simulink model "Simple_Model_Packaging_4_1"  (R2022b)
settings: Solver=VariableStepAuto  StartTime=0.0  StopTime=0.03  RelTol=1e-3
InitFcn:
  | Parameter_Initialize_4
undefined symbols (not defined in the file or in its folder): gcbh, model, rcfiltgaincompat, rsgenpoly
libraries: dspobslib x11, commdigbbndpm3 x6, commdigbbndam3 x6, simulink x5, commblkintrlv2 x4, commfilt2 x4, commsynccomp2 x3, commblkcod2 x2, commrandsrc3 x2, commseqgen3 x2, commchan3 x1, dspsigops x1
(part 2 of 2)

== system Simple_Model_Packaging_4_1/帧序列识别器/Subsystem2 ==
  In1 : Inport
  Constant : Constant
  Constant1 : Constant  Value=-1
  If : If  IfExpression=u1 ==1
  If Action Subsystem : Subsystem  TreatAsAtomicUnit=on
  If Action Subsystem1 : Subsystem  TreatAsAtomicUnit=on
  Merge : Merge
  Out1 : Outport
  wires:
  If Action Subsystem1/1(Out1) -> Merge/2
  If/2 -> If Action Subsystem1/Action
  In1/1 -> If/1
  If Action Subsystem/1(Out1) -> Merge/1
  If/1 -> If Action Subsystem/Action
  Merge/1 -> Out1/1
  Constant1/1 -> If Action Subsystem1/1(In1)
  Constant/1 -> If Action Subsystem/1(In1)

== system Simple_Model_Packaging_4_1/帧序列识别器/Subsystem3 ==
  In1 : Inport
  Constant : Constant
  Constant1 : Constant  Value=-1
  If : If  IfExpression=u1 ==2
  If Action Subsystem : Subsystem  TreatAsAtomicUnit=on
  If Action Subsystem1 : Subsystem  TreatAsAtomicUnit=on
  Merge : Merge
  Out1 : Outport
  wires:
  Constant/1 -> If Action Subsystem/1(In1)
  Constant1/1 -> If Action Subsystem1/1(In1)
  Merge/1 -> Out1/1
  If/1 -> If Action Subsystem/Action
  If Action Subsystem/1(Out1) -> Merge/1
  In1/1 -> If/1
  If/2 -> If Action Subsystem1/Action
  If Action Subsystem1/1(Out1) -> Merge/2

== system Simple_Model_Packaging_4_1/帧序列识别器/Subsystem4 ==
  In1 : Inport
  Constant : Constant
  Constant1 : Constant  Value=-1
  If : If  IfExpression=u1 ==3
  If Action Subsystem : Subsystem  TreatAsAtomicUnit=on
  If Action Subsystem1 : Subsystem  TreatAsAtomicUnit=on
  Merge : Merge
  Out1 : Outport
  wires:
  If Action Subsystem1/1(Out1) -> Merge/2
  If/2 -> If Action Subsystem1/Action
  In1/1 -> If/1
  If Action Subsystem/1(Out1) -> Merge/1
  If/1 -> If Action Subsystem/Action
  Merge/1 -> Out1/1
  Constant1/1 -> If Action Subsystem1/1(In1)
  Constant/1 -> If Action Subsystem/1(In1)

== system Simple_Model_Packaging_4_1/帧序列识别器/Subsystem5 ==
  In1 : Inport
  Constant : Constant
  Constant1 : Constant  Value=-1
  If : If  IfExpression=u1 ==2
  If Action Subsystem : Subsystem  TreatAsAtomicUnit=on
  If Action Subsystem1 : Subsystem  TreatAsAtomicUnit=on
  Merge : Merge
  Out1 : Outport
  wires:
  Constant/1 -> If Action Subsystem/1(In1)
  Constant1/1 -> If Action Subsystem1/1(In1)
  Merge/1 -> Out1/1
  If/1 -> If Action Subsystem/Action
  If Action Subsystem/1(Out1) -> Merge/1
  In1/1 -> If/1
  If/2 -> If Action Subsystem1/Action
  If Action Subsystem1/1(Out1) -> Merge/2

== system Simple_Model_Packaging_4_1/帧序列识别器/Subsystem6 ==
  In1 : Inport
  Constant : Constant
  Constant1 : Constant  Value=-1
  If : If  IfExpression=u1 ==1
  If Action Subsystem : Subsystem  TreatAsAtomicUnit=on
  If Action Subsystem1 : Subsystem  TreatAsAtomicUnit=on
  Merge : Merge
  Out1 : Outport
  wires:
  If Action Subsystem1/1(Out1) -> Merge/2
  If/2 -> If Action Subsystem1/Action
  In1/1 -> If/1
  If Action Subsystem/1(Out1) -> Merge/1
  If/1 -> If Action Subsystem/Action
  Merge/1 -> Out1/1
  Constant1/1 -> If Action Subsystem1/1(In1)
  Constant/1 -> If Action Subsystem/1(In1)

== system Simple_Model_Packaging_4_1/帧序列识别器/Subsystem7 ==
  In1 : Inport
  Constant : Constant
  Constant1 : Constant  Value=-1
  If : If  IfExpression=u1 ==3
  If Action Subsystem : Subsystem  TreatAsAtomicUnit=on
  If Action Subsystem1 : Subsystem  TreatAsAtomicUnit=on
  Merge : Merge
  Out1 : Outport
  wires:
  Constant/1 -> If Action Subsystem/1(In1)
  Constant1/1 -> If Action Subsystem1/1(In1)
  Merge/1 -> Out1/1
  If/1 -> If Action Subsystem/Action
  If Action Subsystem/1(Out1) -> Merge/1
  In1/1 -> If/1
  If/2 -> If Action Subsystem1/Action
  If Action Subsystem1/1(Out1) -> Merge/2

== system Simple_Model_Packaging_4_1/帧序列识别器/Triggered Subsystem ==
  y3_SS : Inport
  Trigger : TriggerPort  TriggerType=falling  VariantControl=(inherit)
  Out1 : Outport
  wires:
  y3_SS/1 -> Out1/1

== system Simple_Model_Packaging_4_1/信源基带解调/Baseband Signal Selector Rx/If Action Subsystem1 ==
  In1 : Inport
  Action Port : ActionPort  ActionPortLabel=elseif(u1 == 2)
  M-PSK Demodulator Baseband : commdigbbndpm3/M-PSK Demodulator Baseband  M=model.user_defined.Rectangular_QAM_Modulator_Baseband.M_Number  OutType=Integer  DecType=Hard decision  VarSource=Dialog  Variance=1  Dec=Gray  Mapping=[0:7]  Ph=0  outDtype1=Inherit via internal rule  outDtype2=Inherit via internal rule  derotateFactorWordLen=16  derotateFactorDataTypeStr=Inherit: Same word length as input  derotateFactorLastDataTypeStr=Inherit: Same word length as input
  Out1 : Outport
  wires:
  In1/1 -> M-PSK Demodulator Baseband/1
  M-PSK Demodulator Baseband/1 -> Out1/1  "REData"

== system Simple_Model_Packaging_4_1/信源基带解调/Baseband Signal Selector Rx/If Action Subsystem4 ==
  In1 : Inport
  Action Port : ActionPort  ActionPortLabel=if(u1 == 1)
  Rectangular QAM Demodulator Baseband : commdigbbndam3/Rectangular QAM Demodulator Baseband  M=model.user_defined.Rectangular_QAM_Modulator_Baseband.M_Number  OutType=Integer  DecType=Hard decision  VarSource=Dialog  Variance=1  Dec=Gray  Mapping=[0:15]  PowType=Min. distance between symbols  MinDist=model.parameter.Rectangular_QAM_Demodulator_Baseband.Minimum_distance  AvgPow=1  PeakPow=1  Ph=0  outDtype1=Inherit via internal rule  outDtype2=Inherit via internal rule  derotateFactorWordLen=16  derotateFactorDataTypeStr=Inherit: Same word length as input  derotateFactorLastDataTypeStr=Inherit: Same word length as input  denormFactorWordLen=16  denormFactorDataTypeStr=Inherit: Same word length as input  denormFactorLastDataTypeStr=Inherit: Same word length as input  prodOutWordLen=32  prodOutOverflowMode=Wrap  prodOutRoundingMode=Floor  prodOutOvFlMode=off  prodOutOvFlModeLastStrValue=off  sumWordLen=32
  Out1 : Outport
  wires:
  In1/1 -> Rectangular QAM Demodulator Baseband/1
  Rectangular QAM Demodulator Baseband/1 -> Out1/1  "REData"

== system Simple_Model_Packaging_4_1/信源基带解调/Baseband Signal Selector Rx/If Action Subsystem5 ==
  In1 : Inport
  Action Port : ActionPort  ActionPortLabel=else
  Rectangular QAM Demodulator Baseband : commdigbbndam3/Rectangular QAM Demodulator Baseband  M=model.user_defined.Rectangular_QAM_Modulator_Baseband.M_Number  OutType=Integer  DecType=Hard decision  VarSource=Dialog  Variance=1  Dec=Gray  Mapping=[0:15]  PowType=Min. distance between symbols  MinDist=2  AvgPow=1  PeakPow=1  Ph=0  outDtype1=Inherit via internal rule  outDtype2=Inherit via internal rule  derotateFactorWordLen=16  derotateFactorDataTypeStr=Inherit: Same word length as input  derotateFactorLastDataTypeStr=Inherit: Same word length as input  denormFactorWordLen=16  denormFactorDataTypeStr=Inherit: Same word length as input  denormFactorLastDataTypeStr=Inherit: Same word length as input  prodOutWordLen=32  prodOutOverflowMode=Wrap  prodOutRoundingMode=Floor  prodOutOvFlMode=off  prodOutOvFlModeLastStrValue=off  sumWordLen=32
  Out1 : Outport
  wires:
  In1/1 -> Rectangular QAM Demodulator Baseband/1
  Rectangular QAM Demodulator Baseband/1 -> Out1/1

== system Simple_Model_Packaging_4_1/信源部分基带调制/Baseband Signal Selector Tx/If Action Subsystem1 ==
  In1 : Inport
  Action Port : ActionPort  ActionPortLabel=elseif(u1 == 2)
  M-PSK Modulator Baseband : commdigbbndpm3/M-PSK Modulator Baseband  M=model.user_defined.Rectangular_QAM_Modulator_Baseband.M_Number  InType=Integer  Enc=Gray  Mapping=[0:7]  Ph=0  outDtype=double  outWordLen=16  outUDDataType=sfix(16)  outFracLenMode=Best precision  outFracLen=15  outDataTypeStr=double  outLastDataTypeStr=double
  Out1 : Outport
  wires:
  M-PSK Modulator Baseband/1 -> Out1/1
  In1/1 -> M-PSK Modulator Baseband/1

== system Simple_Model_Packaging_4_1/信源部分基带调制/Baseband Signal Selector Tx/If Action Subsystem4 ==
  In1 : Inport
  Action Port : ActionPort  ActionPortLabel=if(u1 == 1)
  Rectangular QAM Modulator Baseband : commdigbbndam3/Rectangular QAM Modulator Baseband  M=model.user_defined.Rectangular_QAM_Modulator_Baseband.M_Number  InType=Integer  Enc=Gray  Mapping=[0:15]  PowType=Min. distance between symbols  MinDist=model.parameter.Rectangular_QAM_Modulator_Baseband.Minimum_distance  AvgPow=1  PeakPow=1  Ph=0  outDtype=double  outWordLen=16  outUDDataType=sfix(16)  outFracLenMode=Best precision  outFracLen=15  outDataTypeStr=double  outLastDataTypeStr=double
      settings: LibrarySourceBlock=|
      | commhdldigbbndam/Rectangular QAM
      | Modulator
      | Baseband
  Out1 : Outport
  wires:
  Rectangular QAM Modulator Baseband/1 -> Out1/1
  In1/1 -> Rectangular QAM Modulator Baseband/1

== system Simple_Model_Packaging_4_1/信源部分基带调制/Baseband Signal Selector Tx/If Action Subsystem5 ==
  In1 : Inport
  Action Port : ActionPort  ActionPortLabel=else
  Rectangular QAM Modulator Baseband1 : commdigbbndam3/Rectangular QAM Modulator Baseband  M=model.user_defined.Rectangular_QAM_Modulator_Baseband.M_Number  InType=Integer  Enc=Gray  Mapping=[0:15]  PowType=Min. distance between symbols  MinDist=2  AvgPow=1  PeakPow=1  Ph=0  outDtype=double  outWordLen=16  outUDDataType=sfix(16)  outFracLenMode=Best precision  outFracLen=15  outDataTypeStr=double  outLastDataTypeStr=double
      settings: LibrarySourceBlock=|
      | commhdldigbbndam/Rectangular QAM
      | Modulator
      | Baseband
  Out1 : Outport
  wires:
  In1/1 -> Rectangular QAM Modulator Baseband1/1
  Rectangular QAM Modulator Baseband1/1 -> Out1/1

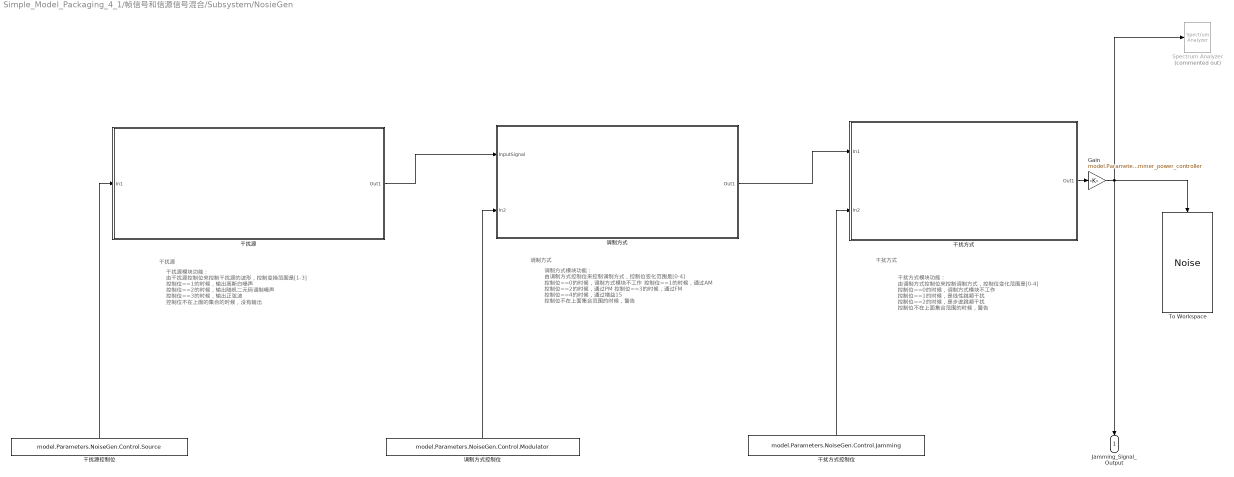
== system Simple_Model_Packaging_4_1/帧信号和信源信号混合/Subsystem/NosieGen ==
  note: 干扰方式模块功能：
      | 由调制方式控制位来控制调制方式，控制位变化范围是[0-4]
      | 控制位==0的时候，调制方式模块不工作
      | 控制位==1的时候，是线性跳频干扰
      | 控制位==2的时候，是步进跳频干扰
      | 控制位不在上面集合范围的时候，警告
  note: 干扰源模块功能：
      | 由干扰源控制位来控制干扰源的波形，控制变换范围是[1-3]
      | 控制位==1的时候，输出高斯白噪声
      | 控制位==2的时候，输出随机二元码调制噪声
      | 控制位==3的时候，输出正弦波
      | 控制位不在上面的集合的时候，没有输出
  note: 调制方式模块功能：
      | 由调制方式控制位来控制调制方式，控制位变化范围是[0-4]
      | 控制位==0的时候，调制方式模块不工作
      | 控制位==1的时候，通过AM
      | 控制位==2的时候，通过PM
      | 控制位==3的时候，通过FM
      | 控制位==4的时候，通过增益15
      | 控制位不在上面集合范围的时候，警告
  note: 干扰方式
  note: 干扰源
  note: 调制方式
  Gain : Gain  Gain=model.Parameters.jammer_power_controller
  Spectrum Analyzer : SpectrumAnalyzer  Commented=on
  To Workspace : ToWorkspace  VariableName=Noise  SaveFormat=Timeseries  SampleTime=-1
  干扰方式 : Subsystem
  干扰方式控制位 : Constant  Value=model.Parameters.NoiseGen.Control.Jamming  SampleTime=Inf
  干扰源 : Subsystem
  干扰源控制位 : Constant  Value=model.Parameters.NoiseGen.Control.Source  SampleTime=Inf
  调制方式 : Subsystem
  调制方式控制位 : Constant  Value=model.Parameters.NoiseGen.Control.Modulator  SampleTime=Inf
  Jamming_Signal_Output : Outport
  wires:
  干扰方式/1(Out1) -> Gain/1
  调制方式/1(Out1) -> 干扰方式/1(In1)
  干扰源/1(Out1) -> 调制方式/1(InputSignal)
  干扰方式控制位/1 -> 干扰方式/2(In2)
  干扰源控制位/1 -> 干扰源/1(In1)
  调制方式控制位/1 -> 调制方式/2(In2)
  Gain/1 -> To Workspace/1, Jamming_Signal_Output/1, Spectrum Analyzer/1

== system Simple_Model_Packaging_4_1/帧序列识别器/Subsystem/If Action Subsystem ==
  In1 : Inport
  Action Port : ActionPort  ActionPortLabel=if(u1 ==0)
  Out1 : Outport
  wires:
  In1/1 -> Out1/1

== system Simple_Model_Packaging_4_1/帧序列识别器/Subsystem/If Action Subsystem1 ==
  In1 : Inport
  Action Port : ActionPort  ActionPortLabel=else
  Out1 : Outport
  wires:
  In1/1 -> Out1/1

== system Simple_Model_Packaging_4_1/帧序列识别器/Subsystem1/If Action Subsystem ==
  In1 : Inport
  Action Port : ActionPort  ActionPortLabel=if(u1 ==3)
  Out1 : Outport
  wires:
  In1/1 -> Out1/1

== system Simple_Model_Packaging_4_1/帧序列识别器/Subsystem1/If Action Subsystem1 ==
  In1 : Inport
  Action Port : ActionPort  ActionPortLabel=else
  Out1 : Outport
  wires:
  In1/1 -> Out1/1

== system Simple_Model_Packaging_4_1/帧序列识别器/Subsystem2/If Action Subsystem ==
  In1 : Inport
  Action Port : ActionPort  ActionPortLabel=if(u1 ==1)
  Out1 : Outport
  wires:
  In1/1 -> Out1/1

== system Simple_Model_Packaging_4_1/帧序列识别器/Subsystem2/If Action Subsystem1 ==
  In1 : Inport
  Action Port : ActionPort  ActionPortLabel=else
  Out1 : Outport
  wires:
  In1/1 -> Out1/1

== system Simple_Model_Packaging_4_1/帧序列识别器/Subsystem3/If Action Subsystem ==
  In1 : Inport
  Action Port : ActionPort  ActionPortLabel=if(u1 ==2)
  Out1 : Outport
  wires:
  In1/1 -> Out1/1

== system Simple_Model_Packaging_4_1/帧序列识别器/Subsystem3/If Action Subsystem1 ==
  In1 : Inport
  Action Port : ActionPort  ActionPortLabel=else
  Out1 : Outport
  wires:
  In1/1 -> Out1/1

== system Simple_Model_Packaging_4_1/帧序列识别器/Subsystem4/If Action Subsystem ==
  In1 : Inport
  Action Port : ActionPort  ActionPortLabel=if(u1 ==3)
  Out1 : Outport
  wires:
  In1/1 -> Out1/1

== system Simple_Model_Packaging_4_1/帧序列识别器/Subsystem4/If Action Subsystem1 ==
  In1 : Inport
  Action Port : ActionPort  ActionPortLabel=else
  Out1 : Outport
  wires:
  In1/1 -> Out1/1

== system Simple_Model_Packaging_4_1/帧序列识别器/Subsystem5/If Action Subsystem ==
  In1 : Inport
  Action Port : ActionPort  ActionPortLabel=if(u1 ==2)
  Out1 : Outport
  wires:
  In1/1 -> Out1/1

== system Simple_Model_Packaging_4_1/帧序列识别器/Subsystem5/If Action Subsystem1 ==
  In1 : Inport
  Action Port : ActionPort  ActionPortLabel=else
  Out1 : Outport
  wires:
  In1/1 -> Out1/1

== system Simple_Model_Packaging_4_1/帧序列识别器/Subsystem6/If Action Subsystem ==
  In1 : Inport
  Action Port : ActionPort  ActionPortLabel=if(u1 ==1)
  Out1 : Outport
  wires:
  In1/1 -> Out1/1

== system Simple_Model_Packaging_4_1/帧序列识别器/Subsystem6/If Action Subsystem1 ==
  In1 : Inport
  Action Port : ActionPort  ActionPortLabel=else
  Out1 : Outport
  wires:
  In1/1 -> Out1/1

== system Simple_Model_Packaging_4_1/帧序列识别器/Subsystem7/If Action Subsystem ==
  In1 : Inport
  Action Port : ActionPort  ActionPortLabel=if(u1 ==3)
  Out1 : Outport
  wires:
  In1/1 -> Out1/1

== system Simple_Model_Packaging_4_1/帧序列识别器/Subsystem7/If Action Subsystem1 ==
  In1 : Inport
  Action Port : ActionPort  ActionPortLabel=else
  Out1 : Outport
  wires:
  In1/1 -> Out1/1

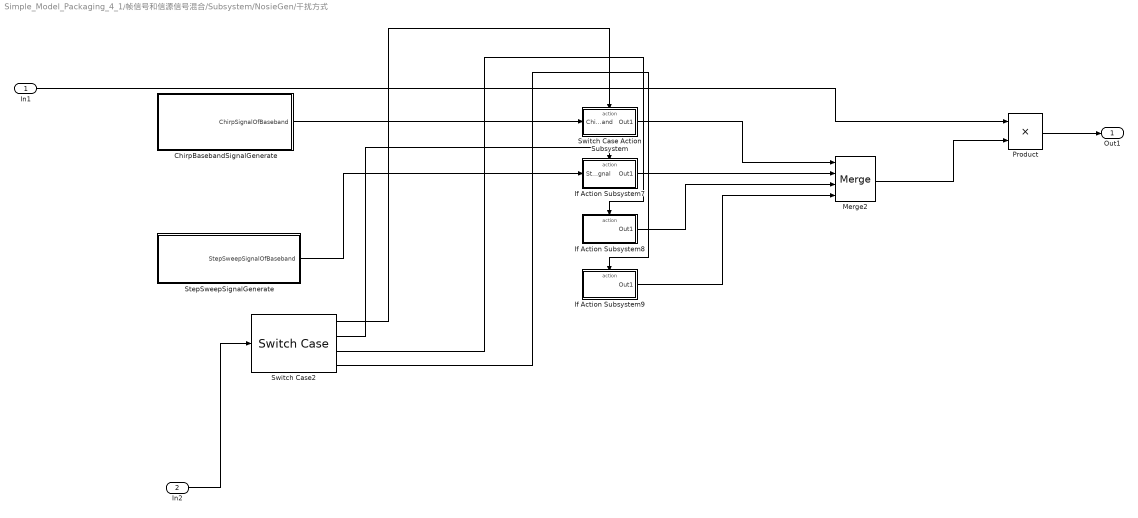
== system Simple_Model_Packaging_4_1/帧信号和信源信号混合/Subsystem/NosieGen/干扰方式 ==
  In1 : Inport
  In2 : Inport  Port=2
  ChirpBasebandSignalGenerate : Subsystem
      settings: AttributesFormatString=|
      | 线性调频模块：线性调频公式(y=exp(2*pi*(f_min*t+0.5*k_chirp*t^2)))
      | 输入参数：
      | 1. f_min,为线性调频信号的起始频率
      | 2.f_max为线性调频信号的终止频率
      | 3.T_chirp为线性调频信号的调频时间
      | 斜率k_sweep = (f_min-f_max)/T_chirp
  If Action Subsystem7 : Subsystem  TreatAsAtomicUnit=on
  If Action Subsystem8 : Subsystem  TreatAsAtomicUnit=on
  If Action Subsystem9 : Subsystem  TreatAsAtomicUnit=on
  Merge2 : Merge  Inputs=4
  Product : Product
  StepSweepSignalGenerate : Subsystem
  Switch Case Action Subsystem : Subsystem  TreatAsAtomicUnit=on
  Switch Case2 : SwitchCase  CaseConditions={1,2,3}
  Out1 : Outport
  wires:
  If Action Subsystem9/1(Out1) -> Merge2/4
  Switch Case Action Subsystem/1(Out1) -> Merge2/1
  If Action Subsystem8/1(Out1) -> Merge2/3
  Switch Case2/3 -> If Action Subsystem8/Action
  Switch Case2/1 -> Switch Case Action Subsystem/Action
  Switch Case2/2 -> If Action Subsystem7/Action
  Switch Case2/4 -> If Action Subsystem9/Action
  ChirpBasebandSignalGenerate/1(ChirpSignalOfBaseband) -> Switch Case Action Subsystem/1(ChirpSignalOfBaseband)
  If Action Subsystem7/1(Out1) -> Merge2/2
  Merge2/1 -> Product/2
  Product/1 -> Out1/1
  In1/1 -> Product/1
  In2/1 -> Switch Case2/1
  StepSweepSignalGenerate/1(StepSweepSignalOfBaseband) -> If Action Subsystem7/1(StepSweepSignal)

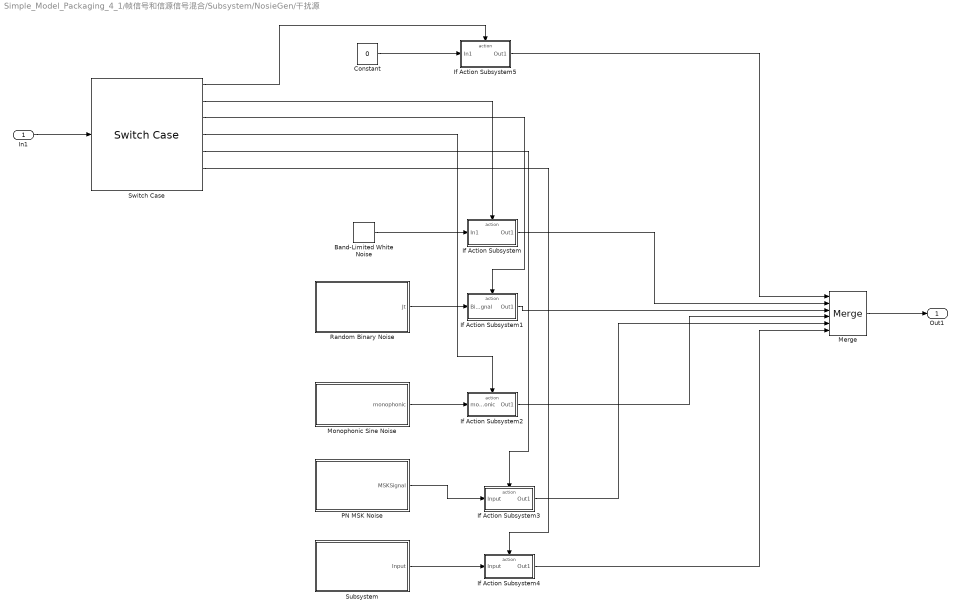
== system Simple_Model_Packaging_4_1/帧信号和信源信号混合/Subsystem/NosieGen/干扰源 ==
  In1 : Inport
  Band-Limited White Noise : simulink/Sources/Band-Limited White Noise  Cov=model.Parameters.NoiseGen.GaussPower  Ts=model.Parameters.NoiseGen.NoiseTs  seed=model.Parameters.NoiseGen.GaussSeed
  Constant : Constant  Value=0  SampleTime=model.Parameters.NoiseGen.NoiseTs
  If Action Subsystem : Subsystem  TreatAsAtomicUnit=on
  If Action Subsystem1 : Subsystem  TreatAsAtomicUnit=on
  If Action Subsystem2 : Subsystem  TreatAsAtomicUnit=on
  If Action Subsystem3 : Subsystem  TreatAsAtomicUnit=on
  If Action Subsystem4 : Subsystem  TreatAsAtomicUnit=on
  If Action Subsystem5 : Subsystem  TreatAsAtomicUnit=on
  Merge : Merge  Inputs=6
  Monophonic Sine Noise : Subsystem
  PN MSK Noise : Subsystem
  Random Binary Noise : Subsystem
  Subsystem : Subsystem
  Switch Case : SwitchCase  CaseConditions={0,1,2,3,4,5}
  Out1 : Outport
  wires:
  Switch Case/3 -> If Action Subsystem1/Action
  If Action Subsystem2/1(Out1) -> Merge/4
  Band-Limited White Noise/1 -> If Action Subsystem/1(In1)
  If Action Subsystem1/1(Out1) -> Merge/3
  Random Binary Noise/1(Jt) -> If Action Subsystem1/1(Binary_Random_Signal)
  Switch Case/4 -> If Action Subsystem2/Action
  Switch Case/2 -> If Action Subsystem/Action
  Merge/1 -> Out1/1
  In1/1 -> Switch Case/1
  Monophonic Sine Noise/1(monophonic) -> If Action Subsystem2/1(monophonic)
  Switch Case/5 -> If Action Subsystem3/Action
  If Action Subsystem3/1(Out1) -> Merge/5
  If Action Subsystem/1(Out1) -> Merge/2
  PN MSK Noise/1(MSKSignal) -> If Action Subsystem3/1(Input)
  Switch Case/6 -> If Action Subsystem4/Action
  Subsystem/1(Input) -> If Action Subsystem4/1(Input)
  If Action Subsystem4/1(Out1) -> Merge/6
  Switch Case/1 -> If Action Subsystem5/Action
  Constant/1 -> If Action Subsystem5/1(In1)
  If Action Subsystem5/1(Out1) -> Merge/1

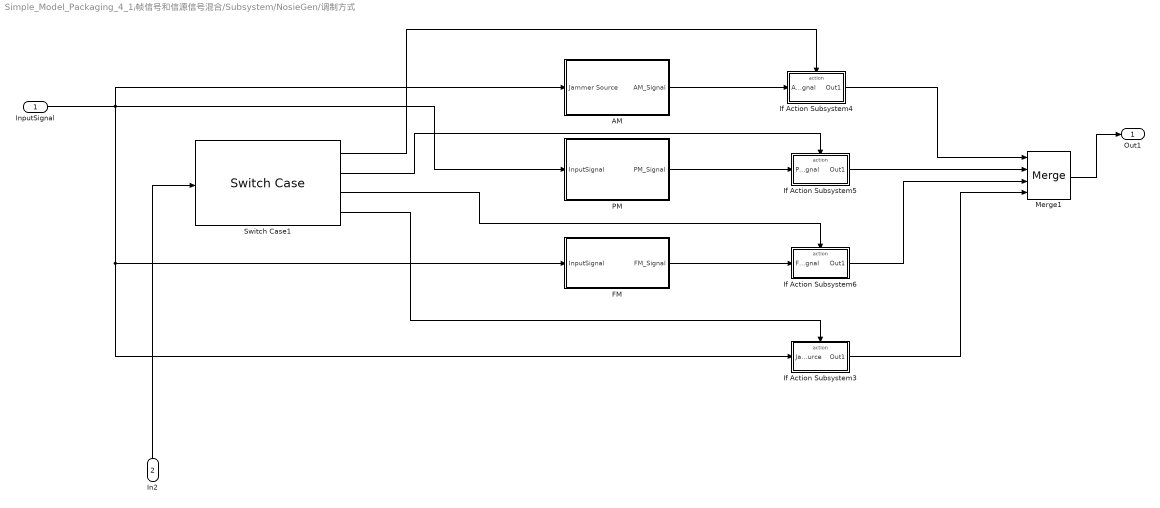
== system Simple_Model_Packaging_4_1/帧信号和信源信号混合/Subsystem/NosieGen/调制方式 ==
  InputSignal : Inport
  In2 : Inport  Port=2
  AM : Subsystem
  FM : Subsystem
  If Action Subsystem3 : Subsystem  TreatAsAtomicUnit=on
  If Action Subsystem4 : Subsystem  TreatAsAtomicUnit=on
  If Action Subsystem5 : Subsystem  TreatAsAtomicUnit=on
  If Action Subsystem6 : Subsystem  TreatAsAtomicUnit=on
  Merge1 : Merge  Inputs=4
  PM : Subsystem
  Switch Case1 : SwitchCase  CaseConditions={1,2,3}
  Out1 : Outport
  wires:
  In2/1 -> Switch Case1/1
  PM/1(PM_Signal) -> If Action Subsystem5/1(PM_Signal)
  Merge1/1 -> Out1/1
  If Action Subsystem3/1(Out1) -> Merge1/4
  If Action Subsystem6/1(Out1) -> Merge1/3
  If Action Subsystem5/1(Out1) -> Merge1/2
  InputSignal/1 -> AM/1(Jammer Source), FM/1(InputSignal), If Action Subsystem3/1(Jammer Source), PM/1(InputSignal)
  AM/1(AM_Signal) -> If Action Subsystem4/1(AM_Signal)
  Switch Case1/2 -> If Action Subsystem5/Action
  Switch Case1/3 -> If Action Subsystem6/Action
  Switch Case1/1 -> If Action Subsystem4/Action
  If Action Subsystem4/1(Out1) -> Merge1/1
  FM/1(FM_Signal) -> If Action Subsystem6/1(FM_Signal)
  Switch Case1/4 -> If Action Subsystem3/Action

== system Simple_Model_Packaging_4_1/帧信号和信源信号混合/Subsystem/NosieGen/干扰方式/ChirpBasebandSignalGenerate ==
  note: 线性调频模块：线性调频公式(y=exp(2*pi*(fmin*t+0.5*k_chirp*t^2)))
      | 输入参数：
      | 1.fmin,为线性调频信号的起始频率
      | 2.fmax为线性调频信号的终止频率
      | 3.T_chirp为线性调频信号的调频时间
      | 斜率k_sweep = (f_min-f_max)/T_chirp
  note: 线性调频模块
  Chirp_Signal_Generation : MATLAB Function  TreatAsAtomicUnit=on
  Constant : Constant  Value=model.Parameters.NoiseGen.Jamming.LinearSweepFmin
  Constant1 : Constant  Value=model.Parameters.NoiseGen.Jamming.LinearSweepT
  Constant2 : Constant  Value=model.Parameters.NoiseGen.Jamming.LinearSweepK
  Digital Clock : DigitalClock  SampleTime=model.Parameters.NoiseGen.NoiseTs
  Frequency_Check : Subsystem  Commented=on
  ChirpSignalOfBaseband : Outport
  wires:
  Digital Clock/1 -> Chirp_Signal_Generation/1(t)
  Chirp_Signal_Generation/1(y) -> ChirpSignalOfBaseband/1  "ChirpSignal"
  Frequency_Check/1(FrequencyConversionLine) -> ?
  Constant/1 -> Chirp_Signal_Generation/2(f_chirp_min)
  Constant2/1 -> Chirp_Signal_Generation/4(k_chirp)
  Constant1/1 -> Chirp_Signal_Generation/3(T_chirp)

== system Simple_Model_Packaging_4_1/帧信号和信源信号混合/Subsystem/NosieGen/干扰方式/If Action Subsystem7 ==
  StepSweepSignal : Inport
  Action Port : ActionPort  ActionPortLabel=case [ 2 ]:
  Out1 : Outport
  wires:
  StepSweepSignal/1 -> Out1/1

== system Simple_Model_Packaging_4_1/帧信号和信源信号混合/Subsystem/NosieGen/干扰方式/If Action Subsystem8 ==
  Action Port : ActionPort  ActionPortLabel=case [ 3 ]:
  Constant : Constant  Value=10
  Constant1 : Constant  Value=0
  Real-Imag to Complex : RealImagToComplex
  Out1 : Outport
  wires:
  Constant/1 -> Real-Imag to Complex/1
  Real-Imag to Complex/1 -> Out1/1
  Constant1/1 -> Real-Imag to Complex/2

== system Simple_Model_Packaging_4_1/帧信号和信源信号混合/Subsystem/NosieGen/干扰方式/If Action Subsystem9 ==
  Action Port : ActionPort  ActionPortLabel=default:
  Constant : Constant
  Constant1 : Constant  Value=0
  Real-Imag to Complex : RealImagToComplex
  Out1 : Outport
  wires:
  Constant/1 -> Real-Imag to Complex/1
  Real-Imag to Complex/1 -> Out1/1
  Constant1/1 -> Real-Imag to Complex/2

== system Simple_Model_Packaging_4_1/帧信号和信源信号混合/Subsystem/NosieGen/干扰方式/StepSweepSignalGenerate ==
  note: 步进调频模块
  Constant : Constant  Value=model.Parameters.NoiseGen.NoiseTs
  Constant1 : Constant  Value=model.Parameters.NoiseGen.Jamming.LinearSweepFmin
  Constant2 : Constant  Value=model.Parameters.NoiseGen.Jamming.StepSweepT
  Constant3 : Constant  Value=model.Parameters.NoiseGen.Jamming.StepSweepDeltaFstep
  Constant4 : Constant  Value=model.Parameters.NoiseGen.Jamming.StepSweepTDwell
  Constant5 : Constant  Value=model.Parameters.NoiseGen.Jamming.StepSweepN
  Digital Clock : DigitalClock  SampleTime=model.Parameters.NoiseGen.NoiseTs
  StepSweep_Signal : MATLAB Function  TreatAsAtomicUnit=on
  StepSweepSignalOfBaseband : Outport
  wires:
  Digital Clock/1 -> StepSweep_Signal/1(t)
  StepSweep_Signal/1(y) -> StepSweepSignalOfBaseband/1  "StepSweepSignal"
  Constant/1 -> StepSweep_Signal/6(Ts)
  Constant1/1 -> StepSweep_Signal/2(f_stepSweep_min)
  Constant2/1 -> StepSweep_Signal/3(T_stepSweep)
  Constant3/1 -> StepSweep_Signal/4(delta_f_stepSweep)
  Constant4/1 -> StepSweep_Signal/5(T_stepSweep_dwell)

== system Simple_Model_Packaging_4_1/帧信号和信源信号混合/Subsystem/NosieGen/干扰方式/Switch Case Action Subsystem ==
  ChirpSignalOfBaseband : Inport
  Action Port : ActionPort  ActionPortLabel=case [ 1 ]:
  Out1 : Outport
  wires:
  ChirpSignalOfBaseband/1 -> Out1/1

== system Simple_Model_Packaging_4_1/帧信号和信源信号混合/Subsystem/NosieGen/干扰源/If Action Subsystem ==
  In1 : Inport
  Action Port : ActionPort  ActionPortLabel=case [ 1 ]:
  Out1 : Outport
  wires:
  In1/1 -> Out1/1

== system Simple_Model_Packaging_4_1/帧信号和信源信号混合/Subsystem/NosieGen/干扰源/If Action Subsystem1 ==
  Binary_Random_Signal : Inport
  Action Port : ActionPort  ActionPortLabel=case [ 2 ]:
  Out1 : Outport
  wires:
  Binary_Random_Signal/1 -> Out1/1

== system Simple_Model_Packaging_4_1/帧信号和信源信号混合/Subsystem/NosieGen/干扰源/If Action Subsystem2 ==
  monophonic : Inport
  Action Port : ActionPort  ActionPortLabel=case [ 3 ]:
  Out1 : Outport
  wires:
  monophonic/1 -> Out1/1

== system Simple_Model_Packaging_4_1/帧信号和信源信号混合/Subsystem/NosieGen/干扰源/If Action Subsystem3 ==
  Input : Inport
  Action Port : ActionPort  ActionPortLabel=case [ 4 ]:
  Out1 : Outport
  wires:
  Input/1 -> Out1/1

== system Simple_Model_Packaging_4_1/帧信号和信源信号混合/Subsystem/NosieGen/干扰源/If Action Subsystem4 ==
  Input : Inport
  Action Port : ActionPort  ActionPortLabel=case [ 5 ]:
  Out1 : Outport
  wires:
  Input/1 -> Out1/1

== system Simple_Model_Packaging_4_1/帧信号和信源信号混合/Subsystem/NosieGen/干扰源/If Action Subsystem5 ==
  In1 : Inport
  Action Port : ActionPort  ActionPortLabel=case [ 0 ]:
  Out1 : Outport
  wires:
  In1/1 -> Out1/1

== system Simple_Model_Packaging_4_1/帧信号和信源信号混合/Subsystem/NosieGen/干扰源/Monophonic Sine Noise ==
  Constant : Constant  Value=model.Parameters.NoiseGen.SineNoisePhi0
  Constant1 : Constant  Value=model.Parameters.NoiseGen.SineNoiseF
  Constant2 : Constant  Value=model.Parameters.NoiseGen.SineNoiseA
  Digital Clock : DigitalClock  SampleTime=model.Parameters.NoiseGen.NoiseTs
  Monophonic_Generate : MATLAB Function  TreatAsAtomicUnit=on
  monophonic : Outport
  wires:
  Digital Clock/1 -> Monophonic_Generate/1(t)
  Constant/1 -> Monophonic_Generate/4(phi0)
  Constant2/1 -> Monophonic_Generate/2(A)
  Constant1/1 -> Monophonic_Generate/3(freq)
  Monophonic_Generate/1(monophonic) -> monophonic/1

== system Simple_Model_Packaging_4_1/帧信号和信源信号混合/Subsystem/NosieGen/干扰源/PN MSK Noise ==
  note: MSK模块
  note: MSK模块：
      | MSK的公式: y = exp(2*pi*fc*t+pi*ak*t/(2Ts)+phi_k)
      | 输入参数：
      | 1. fc:为MSK的中心频率
      | 2. ak:为MSK的第k码元值，数值[-1或者+1]
      | 3. Ts:为MSK的码元周期
      | 4. phi_k:为MSK的第k个码元的修正相位
      | 5. phi_0:为MSK的初始相位
  Buffer : Buffer  N=1  OutputFrames=off
  Complex to Real-Imag : ComplexToRealImag
  Constant : Constant  Value=model.Parameters.NoiseGen.PNMSKF
  Digital Clock : DigitalClock  SampleTime=model.Parameters.NoiseGen.NoiseTs
  MSK Modulator Baseband : commdigbbndcpm2/MSK Modulator Baseband  inputType=Integer  phaseOffset=model.Parameters.NoiseGen.PNMSKPhi0  samplesPerSymbol=model.Parameters.NoiseGen.PNMSKM  RateOptions=Enforce single-rate processing  outDataType=double
  PN Sequence Generator : commseqgen3/PN Sequence Generator  poly=model.Parameters.NoiseGen.PNMSKPolynomial  ini_sta=model.Parameters.NoiseGen.PNMSKInitialstate  outBitMaskSource=Dialog parameter  shift=0  outVarSiz=off  maxOutSizeMode=Dialog parameter  maxOutSize=[10 1]  Ts=model.Parameters.NoiseGen.PNMSKM * model.Parameters.NoiseGen.NoiseTs  sampPerFrame=1  reset=off  bitPackedOutputs=off  outDataType=double  numPackedBits=8  bitPackDataSigned=off  bitPackedOutDType=double
      settings: LibrarySourceBlock=|
      | commhdlsource/PN Sequence
      | Generator
  Random Binary Modulation : MATLAB Function  TreatAsAtomicUnit=on
  Unipolar to Bipolar Converter1 : commutil2/Unipolar to Bipolar Converter  M=2  polarity=Positive  dataType=Inherit via internal rule
  MSKSignal : Outport  OutDataTypeStr=double
  wires:
  Digital Clock/1 -> Random Binary Modulation/2(t)
  Unipolar to Bipolar Converter1/1 -> MSK Modulator Baseband/1
  PN Sequence Generator/1 -> Unipolar to Bipolar Converter1/1
  Constant/1 -> Random Binary Modulation/3(freq)
  MSK Modulator Baseband/1 -> Buffer/1  "cita_k"
  Buffer/1 -> Random Binary Modulation/1(cita_k)
  Random Binary Modulation/1(MSKSignal) -> Complex to Real-Imag/1
  Complex to Real-Imag/1 -> MSKSignal/1

== system Simple_Model_Packaging_4_1/帧信号和信源信号混合/Subsystem/NosieGen/干扰源/Random Binary Noise ==
  note: 改模块采用的是概率为贝努利分布的随机二进制数，随机二元码调制噪声的公式如下：
      | Jt = Am*Jn*cos(2*pi*fj*t+phi0)
      | 本质上是数字调相信号，相位翻转180°
  note: 随机二进制调制噪声
  Bernoulli Binary Generator : commrandsrc3/Bernoulli Binary Generator  ProbabilityOfZero=0.5  SeedSource=Auto  Seed=0  SampleTime=model.Parameters.NoiseGen.NoiseTs  SamplesPerFrame=1  OutputDataType=double  SimulateUsing=Interpreted execution
  Constant : Constant  Value=model.Parameters.NoiseGen.RandBPFA
  Constant1 : Constant  Value=model.Parameters.NoiseGen.RandBPFF
  Constant2 : Constant  Value=model.Parameters.NoiseGen.RandBPFPhi0
  Digital Clock : DigitalClock  SampleTime=model.Parameters.NoiseGen.NoiseTs
  Random Binary Modulation : MATLAB Function  TreatAsAtomicUnit=on
  Unipolar to bipolar : MATLAB Function  TreatAsAtomicUnit=on
  Jt : Outport
  wires:
  Unipolar to bipolar/1(Jn) -> Random Binary Modulation/1(Jn)
  Bernoulli Binary Generator/1 -> Unipolar to bipolar/1(u)
  Random Binary Modulation/1(Jt) -> Jt/1
  Digital Clock/1 -> Random Binary Modulation/2(t)
  Constant/1 -> Random Binary Modulation/3(A)
  Constant1/1 -> Random Binary Modulation/4(freq)
  Constant2/1 -> Random Binary Modulation/5(phi0)

== system Simple_Model_Packaging_4_1/帧信号和信源信号混合/Subsystem/NosieGen/干扰源/Subsystem ==
  Band-Limited White Noise : simulink/Sources/Band-Limited White Noise  Cov=model.Parameters.NoiseGen.RFNoisePower  Ts=model.Parameters.NoiseGen.NoiseTs  seed=model.Parameters.NoiseGen.RFNoiseSeed
  Filter : dsparch4/Biquad Filter  Tag=BlockMethodSubSystem  FilterSource=Filter object  CoeffSource=Specify via dialog  FilterObject=model.Parameters.NoiseGen.RFNoiseFilterObj  IIRFiltStruct=Direct form II  BiQuadCoeffs=[1 2 1 1 -1.48178412853867569 0.831585910854089061;1 2 1 1 -1.27721148327892942 0.578720214976092495;1 2 1 1 -1.14298050253990113 0.412801598096188771;1 2 1 1 -1.06189684687510177 0.31257668783031084;1 2 1 1 -1.02371666858405952 0.265383392069520774]  ScaleValues=[0.0874504455788533558;0.0753771829242907976;0.0674552738890718956;0.0626699602388022664;0.0604166808713653344;1]  IC=0  ICnum=0  ICden=0  a0Flag=Warning  optimizeScaleValues=on  ScaleValueMode=Specify via input port (g)  roundingMode=Floor  overflowMode=off  scaleValueFracLength=14  denProdOutputFracLength=30  denAccumFracLength=30  secondMemoryFracLength=15
  Input : Outport
  wires:
  Band-Limited White Noise/1 -> Filter/1
  Filter/1 -> Input/1

== system Simple_Model_Packaging_4_1/帧信号和信源信号混合/Subsystem/NosieGen/调制方式/AM ==
  Jammer Source : Inport
  AM_Carrier : MATLAB Function  TreatAsAtomicUnit=on
  Constant : Constant  Value=model.Parameters.NoiseGen.Modulator.AMA
  Constant1 : Constant  Value=model.Parameters.NoiseGen.Modulator.AMF
  Constant2 : Constant  Value=model.Parameters.NoiseGen.Modulator.Ma
  Digital Clock : DigitalClock  SampleTime=model.Parameters.NoiseGen.NoiseTs
  AM_Signal : Outport
  wires:
  Digital Clock/1 -> AM_Carrier/1(t)
  AM_Carrier/1(y) -> AM_Signal/1  "ChirpSignal"
  Constant2/1 -> AM_Carrier/5(Ma)
  Constant1/1 -> AM_Carrier/3(freq)
  Constant/1 -> AM_Carrier/2(A)
  Jammer Source/1 -> AM_Carrier/4(carrier_low_freq)

== system Simple_Model_Packaging_4_1/帧信号和信源信号混合/Subsystem/NosieGen/调制方式/FM ==
  InputSignal : Inport
  Constant : Constant  Value=model.Parameters.NoiseGen.Modulator.FMA
  Constant1 : Constant  Value=model.Parameters.NoiseGen.Modulator.FMF
  Constant2 : Constant  Value=model.Parameters.NoiseGen.Modulator.FMPhi0
  Constant3 : Constant  Value=model.Parameters.NoiseGen.Modulator.FMK
  Digital Clock : DigitalClock  SampleTime=model.Parameters.NoiseGen.NoiseTs
  MATLAB Function : MATLAB Function  TreatAsAtomicUnit=on
  FM_Signal : Outport
  wires:
  Digital Clock/1 -> MATLAB Function/1(t)
  MATLAB Function/1(y) -> FM_Signal/1
  InputSignal/1 -> MATLAB Function/2(signal)
  Constant/1 -> MATLAB Function/3(A)
  Constant1/1 -> MATLAB Function/4(freq)
  Constant2/1 -> MATLAB Function/5(phi0)
  Constant3/1 -> MATLAB Function/6(K)

== system Simple_Model_Packaging_4_1/帧信号和信源信号混合/Subsystem/NosieGen/调制方式/If Action Subsystem3 ==
  Jammer Source : Inport
  Action Port : ActionPort  ActionPortLabel=default:
  Out1 : Outport
  wires:
  Jammer Source/1 -> Out1/1

== system Simple_Model_Packaging_4_1/帧信号和信源信号混合/Subsystem/NosieGen/调制方式/If Action Subsystem4 ==
  AM_Signal : Inport
  Action Port : ActionPort  ActionPortLabel=case [ 1 ]:
  Out1 : Outport
  wires:
  AM_Signal/1 -> Out1/1

== system Simple_Model_Packaging_4_1/帧信号和信源信号混合/Subsystem/NosieGen/调制方式/If Action Subsystem5 ==
  PM_Signal : Inport
  Action Port : ActionPort  ActionPortLabel=case [ 2 ]:
  Out1 : Outport
  wires:
  PM_Signal/1 -> Out1/1

== system Simple_Model_Packaging_4_1/帧信号和信源信号混合/Subsystem/NosieGen/调制方式/If Action Subsystem6 ==
  FM_Signal : Inport
  Action Port : ActionPort  ActionPortLabel=case [ 3 ]:
  Out1 : Outport
  wires:
  FM_Signal/1 -> Out1/1

== system Simple_Model_Packaging_4_1/帧信号和信源信号混合/Subsystem/NosieGen/调制方式/PM ==
  InputSignal : Inport
  Constant : Constant  Value=model.Parameters.NoiseGen.Modulator.PMA
  Constant1 : Constant  Value=model.Parameters.NoiseGen.Modulator.PMF
  Constant2 : Constant  Value=model.Parameters.NoiseGen.Modulator.PMPhi0
  Constant3 : Constant  Value=model.Parameters.NoiseGen.Modulator.PMK
  Digital Clock : DigitalClock  SampleTime=model.Parameters.NoiseGen.NoiseTs
  MATLAB Function : MATLAB Function  TreatAsAtomicUnit=on
  PM_Signal : Outport
  wires:
  Digital Clock/1 -> MATLAB Function/1(t)
  InputSignal/1 -> MATLAB Function/2(signal)
  MATLAB Function/1(y) -> PM_Signal/1
  Constant/1 -> MATLAB Function/3(A)
  Constant1/1 -> MATLAB Function/4(freq)
  Constant3/1 -> MATLAB Function/5(K)
  Constant2/1 -> MATLAB Function/6(phi0)

== system Simple_Model_Packaging_4_1/帧信号和信源信号混合/Subsystem/NosieGen/干扰方式/ChirpBasebandSignalGenerate/Frequency_Check ==
  ChirpSignal : Inport
  Derivative : Derivative
  Phase Extractor : dspsigops/Phase Extractor  TreatFramesIndependently=off  SimulateUsing=Code generation
  FrequencyConversionLine : Outport
  wires:
  ChirpSignal/1 -> Phase Extractor/1
  Phase Extractor/1 -> Derivative/1
  Derivative/1 -> FrequencyConversionLine/1

== matlab function Simple_Model_Packaging_4_1/帧信号和信源信号混合/Subsystem/NosieGen/干扰方式/ChirpBasebandSignalGenerate/Chirp_Signal_Generation ==
  data: y output; t input; f_chirp_min input; T_chirp input; k_chirp input
function y = ChirpSignal(t, f_chirp_min, T_chirp, k_chirp)
    t = mod(t,T_chirp);
    y = exp(1i*2*pi*(f_chirp_min*t+0.5*k_chirp*t^2));
end

== matlab function Simple_Model_Packaging_4_1/帧信号和信源信号混合/Subsystem/NosieGen/干扰方式/StepSweepSignalGenerate/StepSweep_Signal ==
  data: y output; t input; f_stepSweep_min input; T_stepSweep input; delta_f_stepSweep input; T_stepSweep_dwell input; Ts input; N_stepSweep input
function y  = StepSweep(t, f_stepSweep_min, T_stepSweep, delta_f_stepSweep, T_stepSweep_dwell, Ts, N_stepSweep)
    a = mod(t,T_stepSweep)+Ts/10000;
    b = fix(a/T_stepSweep_dwell);
    if b == N_stepSweep
        b = N_stepSweep - 1;
    end
    f = (f_stepSweep_min+b*delta_f_stepSweep);
    y = exp(1i*2*pi*f*t);
end

== matlab function Simple_Model_Packaging_4_1/帧信号和信源信号混合/Subsystem/NosieGen/干扰源/Monophonic Sine Noise/Monophonic_Generate ==
  data: t input; A input; freq input; monophonic output; phi0 input
function monophonic = MonophonicGenerate(t, A, freq, phi0)
    monophonic = A * sin(2*pi*freq*t+phi0);
end

== matlab function Simple_Model_Packaging_4_1/帧信号和信源信号混合/Subsystem/NosieGen/干扰源/PN MSK Noise/Random Binary Modulation ==
  data: cita_k input; MSKSignal output; t input; freq input
function MSKSignal = fcn(cita_k,t, freq)
    MSKSignal = cita_k * cos(2*pi*freq*t);
end

== matlab function Simple_Model_Packaging_4_1/帧信号和信源信号混合/Subsystem/NosieGen/干扰源/Random Binary Noise/Random Binary Modulation ==
  data: Jn input; Jt output; t input; A input; freq input; phi0 input
function Jt = fcn(Jn,t,A,freq,phi0)
    Jt = A*Jn*cos(2*pi*freq*t+phi0);
end

== matlab function Simple_Model_Packaging_4_1/帧信号和信源信号混合/Subsystem/NosieGen/干扰源/Random Binary Noise/Unipolar to bipolar ==
  data: u input; Jn output
function Jn= fcn(u)
    Jn = 2*u-1;
end

== matlab function Simple_Model_Packaging_4_1/帧信号和信源信号混合/Subsystem/NosieGen/调制方式/AM/AM_Carrier ==
  data: y output; t input; A input; freq input; carrier_low_freq input; Ma input
function y = AM_Carrier(t, A, freq, carrier_low_freq, Ma)
    y = A*(1+Ma*carrier_low_freq)*cos(2*pi*freq*t);
end

== matlab function Simple_Model_Packaging_4_1/帧信号和信源信号混合/Subsystem/NosieGen/调制方式/FM/MATLAB Function ==
  data: t input; signal input; y output; A input; freq input; phi0 input; K input
function y = FM(t, signal, A, freq, phi0, K)
   y = A*cos(2*pi*(freq+K*signal)*t+phi0) ;
end

== matlab function Simple_Model_Packaging_4_1/帧信号和信源信号混合/Subsystem/NosieGen/调制方式/PM/MATLAB Function ==
  data: t input; signal input; y output; A input; freq input; K input; phi0 input
function y = PM(t, signal, A, freq, K, phi0)
   y = A*cos(2*pi*freq*t+K*signal+phi0) ;
end

== matlab function Simple_Model_Packaging_4_1/本地载波生成模块/MATLAB Function ==
  data: y output; t input; f_chirp_min input; f_chirp_max input; T_chirp input
% function y = carrierGenerator(t)
%     fc = 5e6;
%     y = exp(1i*2*pi*fc*t);

function y = carrierGenerator(t, f_chirp_min, f_chirp_max, T_chirp)
    k_chirp = (f_chirp_max-f_chirp_min)/T_chirp;
    t = mod(t,T_chirp);
    y = exp(1i*2*pi*(f_chirp_min*t+0.5*k_chirp*t^2));

end

== matlab function Simple_Model_Packaging_4_1/帧信号和信源信号混合/发射时序控制 ==
  data: t input; y1_FF output; Frame_Front input; Waveform_Generation_Flag_Transmit data_store_memory; Frame_Back input; y2_FB output; y3_SS output; Signal_Source input; RandomIntegerSignal input; RandomIntegerSignalTimeSelectivity output; FrameSignalSynchronization output; Waveform_Offset input; Waveform_Period input; Frame_Period_Unit_Number input; Frame_Period_Unit_Duration input; Frame_Back_StartPoint_Offset_Control input; Ts input
function [y1_FF, y2_FB, y3_SS, RandomIntegerSignalTimeSelectivity, FrameSignalSynchronization] = timeController(t, Frame_Front, Frame_Back, Signal_Source, RandomIntegerSignal, Waveform_Offset, Waveform_Period, Frame_Period_Unit_Number, Frame_Period_Unit_Duration, Frame_Back_StartPoint_Offset_Control, Ts)
global Waveform_Generation_Flag_Transmit;

Frame_Duration = Frame_Period_Unit_Duration * Frame_Period_Unit_Number;
Frame_Front_StartPoint = mod(t-Waveform_Offset, Waveform_Period);
Frame_Back_StartPoint = mod(t-Waveform_Offset, Waveform_Period) - (Waveform_Period - Frame_Duration - Frame_Back_StartPoint_Offset_Control);
Signal_Source_StartPoint = Frame_Front_StartPoint + Frame_Duration;
Signal_Source_EndPoint = Frame_Back_StartPoint;
Frame_Back_EndPoint = Frame_Back_StartPoint - Frame_Duration;

% global Waveform_Generation_Flag;

% if  ( Frame_Front_StartPoint < Ts/10) || ((Frame_Back_StartPoint > -Ts/10) && (Frame_Back_StartPoint < Ts/10)) || ((Signal_Source_StartPoint>-Ts/10) && (Signal_Source_EndPoint<Ts/10))
if  ( Frame_Front_StartPoint < Ts/100) || ((Frame_Back_StartPoint > -Ts/100) && (Frame_Back_EndPoint < Ts/100)) || ((Signal_Source_StartPoint>-Ts/100) && (Signal_Source_EndPoint<Ts/100))
    Waveform_Generation_Flag_Transmit = int8(1);
end

if Waveform_Generation_Flag_Transmit == int8(1)
    if Frame_Front_StartPoint < Frame_Duration
        y1_FF = Frame_Front;
        y2_FB = complex(0);
        y3_SS = complex(0);
        RandomIntegerSignalTimeSelectivity = 0;
        FrameSignalSynchronization = 0;

    elseif (Frame_Back_StartPoint>=0) && (Frame_Back_StartPoint<Frame_Duration)
        y1_FF = complex(0);
        y2_FB = Frame_Back;
        y3_SS = complex(0);
        RandomIntegerSignalTimeSelectivity = 0;
        FrameSignalSynchronization = 0;

    elseif (Signal_Source_StartPoint>0) && (Signal_Source_EndPoint<0)
        y1_FF = complex(0);
        y2_FB = complex(0);
        y3_SS = Signal_Source;
        RandomIntegerSignalTimeSelectivity = RandomIntegerSignal;
        FrameSignalSynchronization = 1;
    else
        Waveform_Generation_Flag_Transmit = int8(0);
        y1_FF = complex(0);
        y2_FB = complex(0);
        y3_SS = complex(0);
        RandomIntegerSignalTimeSelectivity = 0;
        FrameSignalSynchronization = 0;
    end
else
    y1_FF = complex(0);
    y2_FB = complex(0);
    y3_SS = complex(0);
    RandomIntegerSignalTimeSelectivity = 0;
    FrameSignalSynchronization = 0;
end


end

== matlab function Simple_Model_Packaging_4_1/帧信号和信源信号混合/MATLAB Function2 ==
  data: ReceicedSignal input; t input; y1_FF output; y2_FB output; y3_SS output; Waveform_Generation_Flag_Receive data_store_memory; FrameSignalSynchronization output; Waveform_Offset input; Waveform_Period input; Frame_Period_Unit_Number input; Frame_Period_Unit_Duration input; Frame_Back_StartPoint_Offset_Control input; Ts input
function [y1_FF, y2_FB, y3_SS, FrameSignalSynchronization] = timeSynchronization(ReceicedSignal, t, Waveform_Offset, Waveform_Period, Frame_Period_Unit_Number, Frame_Period_Unit_Duration, Frame_Back_StartPoint_Offset_Control, Ts)
global Waveform_Generation_Flag_Receive;

Frame_Duration = Frame_Period_Unit_Duration * Frame_Period_Unit_Number;
Frame_Front_StartPoint = mod(t-Waveform_Offset, Waveform_Period);
Frame_Back_StartPoint = mod(t-Waveform_Offset, Waveform_Period) - (Waveform_Period - Frame_Duration - Frame_Back_StartPoint_Offset_Control);
Signal_Source_StartPoint = Frame_Front_StartPoint + Frame_Duration;
Signal_Source_EndPoint = Frame_Back_StartPoint;
Frame_Back_EndPoint = Frame_Back_StartPoint - Frame_Duration;


% global Waveform_Generation_Flag;

if  ( Frame_Front_StartPoint < Ts/100) || ((Frame_Back_StartPoint > -Ts/100) && (Frame_Back_EndPoint < Ts/100)) || ((Signal_Source_StartPoint>-Ts/100) && (Signal_Source_EndPoint<Ts/100))
    Waveform_Generation_Flag_Receive = int8(1);
end

if Waveform_Generation_Flag_Receive == int8(1)
    if Frame_Front_StartPoint < Frame_Duration
        y1_FF = ReceicedSignal;
        y2_FB = complex(0);
        y3_SS = complex(0);
        FrameSignalSynchronization = 0;

    elseif (Frame_Back_StartPoint>0) && (Frame_Back_StartPoint<Frame_Duration)
        y1_FF = complex(0);
        y2_FB = ReceicedSignal;
        y3_SS = complex(0);
        FrameSignalSynchronization = 0;

    elseif (Signal_Source_StartPoint>0) && (Signal_Source_EndPoint<0)
        y1_FF = complex(0);
        y2_FB = complex(0);
        y3_SS = ReceicedSignal;
        FrameSignalSynchronization = 1;

    else
        Waveform_Generation_Flag_Receive = int8(0);
        y1_FF = complex(0);
        y2_FB = complex(0);
        y3_SS = complex(0);
        FrameSignalSynchronization = 0;
    end
else
    y1_FF = complex(0);
    y2_FB = complex(0);
    y3_SS = complex(0);
    FrameSignalSynchronization = 0;
end

end

== matlab function Simple_Model_Packaging_4_1/帧信号控制模块/帧信号控制模块 ==
  data: frameRecognition input; Sig_Control_Source output; StartFFCountFlag data_store_memory; Count1 data_store_memory; StartFBCountFlag data_store_memory; Count2 data_store_memory; tirggerTime data_store_memory; lastFrameRecognition data_store_memory; Frame_Period_Unit_Duration input; Ts input
function Sig_Control_Source = frameTimeConrol(frameRecognition, Frame_Period_Unit_Duration, Ts)
global Count1;
global Count2;
global tirggerTime;
global lastFrameRecognition
global StartFFCountFlag
global StartFBCountFlag

if (lastFrameRecognition ==1)&& (frameRecognition == 0)  %当检测到信号下降沿时
    tirggerTime = tirggerTime + int64(1);
    if  ~((Count1==0) && (Count2==0))
        Duration = max(double(Count1)* Ts, double(Count2)* Ts);
        if Duration < Frame_Period_Unit_Duration*4.1    %对触发进行鉴别，若触发时间过短，表明短时内连续存在两个帧信号,需将触发次数减一、两个时间计数器均置零，若为连续两个帧头信号，则将所有标志重置为帧尾状态，计数时间重置，若为连续两个帧尾信号，则将所有标志重置为帧尾状态
            tirggerTime = tirggerTime - int64(1);
            Count1 = uint64(0);
            Count2 = uint64(0);
        end
    end

    if mod(int64(tirggerTime),int64(2)) == 1      %奇数次触发表明为帧头，开始帧头计数、停止帧尾计数并输出高电平控制信号
        StartFFCountFlag = int8(1);
        StartFBCountFlag = int8(0);
    elseif mod(int64(tirggerTime),int64(2)) == 0  %偶数次触发表明为帧尾，停止帧头计数、开始帧尾计数并输出低电平控制信号
        StartFFCountFlag = int8(0);
        StartFBCountFlag = int8(1);
    end
else
    tirggerTime = tirggerTime;
end



if StartFFCountFlag==1    %若帧头标志置位，则开启帧头计数 
    Count1 = Count1 + uint64(1);
    Sig_Control_Source = 1;
else                      %若帧头标志未置位，则关闭帧头计数 
    Count1 = uint64(0);
    Sig_Control_Source = 0;
end

if StartFBCountFlag==1    %若帧尾标志置位，则开启帧尾计数 
    Count2 = Count2 + uint64(1);
else                      %若帧尾标志未置位，则关闭帧尾计数 
    Count2 = uint64(0);
end

lastFrameRecognition = int8(frameRecognition);
end

== matlab function Simple_Model_Packaging_4_1/帧信号基带调制模块/rateTransitionUserDefined ==
  data: y output; input input
% function y = carrierGenerator(t)
%     fc = 5e6;
%     y = exp(1i*2*pi*fc*t);

function y = rateTransition(input)
    p = 10;
    q = 1;
    y = resample(input,p,q);
%     y(1:100) = repmat(y(100),1,100);
%     y(end-99:end) = repmat(y(end-99),1,100);
end

== matlab function Simple_Model_Packaging_4_1/帧信号基带解调/MATLAB Function3 ==
  data: y output; input input
% function y = carrierGenerator(t)
%     fc = 5e6;
%     y = exp(1i*2*pi*fc*t);

function y = rateTransition(input)
    p = 1;
    q = 10;
    y = resample(input,p,q);
%     y(1:10) = repmat(y(10),1,10);
%     y(end-9:end) = repmat(y(end-9),1,10);
end
